simulink model "DR18E_Testpult"  (R2017a)
settings: Solver=ode1  StartTime=0.0  StopTime=Inf  FixedStep=0.001  RelTol=1e-3
PostLoadFcn:
  | , if any(exist('dsrtsu_mdlpostloadfcn', 'file') == [2, 3, 6]), try dsrtsu_mdlpostloadfcn('Execute', bdroot); catch fprintf('Error in PostLoadFcn (dsrtsu_mdlpostloadfcn) for model "%s":\n %s\n', bdroot, lasterr); end, end,
model workspace: external: MATLAB File C:\Users\DeltaRacing\Documents\dSPACE\MABX_DR18E\Model\DR18E_MABX_Parameter.m (data not in the file)
values from neighbouring files (symbols this model uses):
  am = 1/Ts    (= 1)    [DR18E_MABX_Parameter.m]
  bm = K/Ts    (= 0.05)    [DR18E_MABX_Parameter.m]
  cf = 41350    [DR18E_MABX_Parameter.m]
  cr = 41350    [DR18E_MABX_Parameter.m]
  Derating_HV_Battery_Kapa = 1    [DR18E_MABX_Parameter.m]
  Derating_Start_km = 16    [DR18E_MABX_Parameter.m]
  Drive_Mode = 0    [DR18E_MABX_Parameter.m]
  g = 1    [DR18E_MABX_Parameter.m]
  Gas_Modus = 2    [DR18E_MABX_Parameter.m]
  HV_Power_max = 80    [DR18E_MABX_Parameter.m]
  i_Getriebe = 3.3    [DR18E_MABX_Parameter.m]
  i_Lenkgetriebe = 4.32    [DR18E_MABX_Parameter.m]
  K_SET = 1    [DR18E_MABX_Parameter.m]
  Kapazitaet_HV_Battery_kWh = 6.6    [DR18E_MABX_Parameter.m]
  KW_T_Soll = 37    [DR18E_MABX_Parameter.m]
  lf = 1.2    [DR18E_MABX_Parameter.m]
  lr = 1.15    [DR18E_MABX_Parameter.m]
  m = 310    [DR18E_MABX_Parameter.m]
  M_max = 150    [DR18E_MABX_Parameter.m]
  Power_Limit_onoff = 0    [DR18E_MABX_Parameter.m]
  Reifenradius = 0.2351    [DR18E_MABX_Parameter.m]
  Strecke_Endu_km = 22    [DR18E_MABX_Parameter.m]
  TC_Decr_Gas = 0.00005    (= 5e-05)    [DR18E_MABX_Parameter.m]
  TC_Derivative = 0.4    [DR18E_MABX_Parameter.m]
  TC_Incr_Gas = 0.005    [DR18E_MABX_Parameter.m]
  TC_On = 0    [DR18E_MABX_Parameter.m]
  TC_Relay_Off = 0.065    [DR18E_MABX_Parameter.m]
  TC_Relay_On = 0.07    [DR18E_MABX_Parameter.m]
  TV_Mode = 2    [DR18E_MABX_Parameter.m]
  TV_On = 0    [DR18E_MABX_Parameter.m]
  TV_Override = 1    [DR18E_MABX_Parameter.m]
  y = 0.8    [DR18E_MABX_Parameter.m]
undefined symbols (not defined in the file or in its folder): D, DiscIntNeverNeededParam, I, K_OL, P
libraries: simulink x288, rtican x105, rtiusbflightreclib x40, rti1401lib_dio_type3 x10, simulink_extras x10, rti1401lib_adc_type4 x8, rti1401lib_II_base x7
(part 9 of 28)

== system DR18E_Testpult/Eingabe Fahrzeug/Sensorboard Mitte ==
  Bus Creator : BusCreator  Inputs=4
  Bus Creator1 : BusCreator  Inputs=3
  Dashboard_AUX : rtican/RTICAN Receive (RX)   Reserved1=[]  Reserved2=[]  Reserved3=[]  Reserved4=[]  SfcnMessage=[]  Msg_Struct=[]  BoardTypeNo=[]  BoardNo=[]  ChannelNo=[]  Parameters=[]  DialogFcn=[]  UnitName=[]  Revision=[]  UnitValues=[]  DSProperties=struct('RTI',struct('Version',uint32(5),'BlockType',struct('isSLSource',uint8(1),'isSLSink',uint8(1),'isHWSource',uint8(0),'isHWSink',uint8(0),'isSetup',uint8(0),'isInline',uint8(1),'isNonInline',uint8(0),'isInterrupt',uint8(0),'isChannelwise',uint8(0)),'IOBoardType','RTICAN','UnitType','MESSAGE','Identifier','RX','DialogType','MSVC','BlockSet','RTICAN','SlaveProcessor','CAN'))  RTIBlockInterface=struct('OutputPortsWidth',int32([1 1 1 1 1]),'OutputPortsActive',[1 1 1 1 1],'OutputPortsName',{{'Notaus_Cockpit','Crashsensor',['RX status'],['RX time'],['RX delta time']}},'OutputPortsDataType',{{'SS_DOUBLE','SS_DOUBLE','SS_DOUBLE','SS_DOUBLE','SS_DOUBLE'}},'OutputPortsLabel',{{'Notaus_Cockpit','Crashsensor','','',''}},'OutputPortsLabelMode','ON','InputPortsWidth',int32(0),'InputPortsActive',0,'DialogFcn','rtican_message_interface_gui','BlockDisplay',{{'','center'}},'IconTransparency','on','ParameterTunableNames',{{}},'InitLevel',3,'BlockName',struct('Token',{{'Dashboard_AUX'}}),'SampleTime',{{-1}},'TriggerPort',{{'none'}},'EnablePort',{{'none'}})  RTIBlockParameters=struct('BoardTypeNo',{{1,'OFF',[]}},'BoardNo',{{2,'ON',[1 16]}},'ChannelNo',{{1,'ON',[1 2]}},'Parameters',{{struct('DataFileSupport',struct('DataFileSelectedMaster',1,'DataFileSelectedLocal',1,'DataFileName','c:\users\deltaracing\documents\canoe\dr18e\dbc\dr18e.dbc|','DataFileDate',['16-Feb-2019 13:23:09'],'SelectedFile','..\..\..\canoe\dr18e_test\dr18e\dbc\dr18e.dbc','InterfaceFcn','rtican_dbc_file_parser'),'Options',struct('StatusSelected',1,'TimeSelected',1,'DeltaTimeSelected',1,'BytePortSelected',0,'MessageLengthSelected',0,'TriggerPort',struct('Selected',0,'TriggerType',0),'UserCoding',struct('Selected',0,'InterfaceFile','UserDecodingFile','FcnName','UserDecodeFcn','InportSelected',0,'InportWidth',1,'OutportSelected',0,'OutportWidth',1),'EnablePortSelected',0,'SignalOnPortnameSelected',1,'UseRXService',0),'Message',struct('MsgOnBlocknameSelected',1,'MsgName','Dashboard_AUX','MsgIdFormat',0,'MsgId',786,'MsgLength',2,'NumSignals',2,'SampleTime',-1,'Signal',struct('SgnName',{'Notaus_Cockpit','Crashsensor'},'SgnStartBit',{0,8},'SgnLength',{8,8},'ByteLayout',{0,0},'Factor',{1,1},'Offset',{0,0},'SgnComment',{'',''},'SgnUnit',{'',''},'Min',{0,0},'Max',{255,255},'SgnType',{0,0},'SLDataType',{'SS_DOUBLE','SS_DOUBLE'},'DataType',{0,0},'ModeValue',{-1,-1}),'MsgIdNumFormat',0,'MsgComment',{{''}}),'Version',1.2,'general',struct('isFromLib',0)),'OFF',[]}},'GroupId',{{struct('Group',{{'RTICAN'}},'No',1,'Behavior',{{'NAMECHANGE'}},'BlockType',{{'SINK'}},'NameChangeFlag',0),'OFF',[]}},'SFcnRTICANMessage',{{struct('MsgType','RX','SFcnPortType','Scalar','MsgName','Dashboard_AUX','MsgIdFormat','STD','MsgId',786,'MsgLength',2,'NumSignals',2,'SampleTime',-1,'Signal',struct('SgnName',{'Notaus_Cockpit','Crashsensor'},'SgnStartBit',{0,8},'SgnLength',{8,8},'ByteLayout',{['little endian'],['little endian']},'Factor',{1,1},'Offset',{0,0},'SgnType',{'standard','standard'},'SLDataType',{'SS_DOUBLE','SS_DOUBLE'},'DataType',{['unsigned int'],['unsigned int']},'ModeValue',{-1,-1}),'StatusSelected','yes','TimeSelected','yes','DeltaTimeSelected','yes','BytePortSelected','no','MessageLengthSelected','no','TriggerPort',struct('Selected','no','TriggerType',0),'UserCoding',struct('Selected','no','InterfaceFile','UserDecodingFile','FcnName','UserDecodeFcn','InportSelected','no','InportWidth',1,'OutportSelected','no','OutportWidth',1),'EnablePortSelected','no','UseRXService','no','BoardType','DS1','BoardNo',2,'ControllerNo',1),'OFF',[]}},'TLCFileName',{{'rtican_rx_message','OFF',[]}})  RTISFcnParameters=struct('SFcnRTICANMessage','struct','TLCFileName','char')  RTIBlockParaDefault=struct('BoardTypeNo',4302,'BoardNo',1,'ChannelNo',1,'Parameters',struct('DataFileSupport',struct('DataFileSelectedMaster',0,'DataFileSelectedLocal',0,'DataFileName','','DataFileDate','','SelectedFile',['<no file selected>']),'Options',struct('StatusSelected',1,'TimeSelected',1,'DeltaTimeSelected',1,'BytePortSelected',0,'MessageLengthSelected',0,'TriggerPort',struct('Selected',0,'TriggerType','rising'),'UserCoding',struct('Selected',0,'InterfaceFile','UserDecodingFile','FcnName','UserDecodeFcn','InportSelected',0,'InportWidth',1,'OutportSelected',0,'OutportWidth',1),'EnablePortSelected',0,'SignalOnPortnameSelected',1,'UseRXService',0),'Message',struct('MsgOnBlocknameSelected',0,'MsgName',['RX Message'],'MsgIdFormat',0,'MsgId',100,'MsgLength',8,'NumSignals',1,'SampleTime',-1,'Signal',struct('SgnName',['RX signal'],'SgnStartBit',0,'SgnLength',8,'SgnType',0,'ModeValue',-1,'DataType',0,'SLDataType','SS_DOUBLE','ByteLayout',0,'Factor',1,'Offset',0,'Min',0,'Max',255,'SgnComment',{{}},'SgnUnit',''),'MsgIdNumFormat',0,'MsgComment',{{''}}),'Version',1.2,'general',struct('isFromLib',1)),'GroupId',struct('Group',{{'RTICAN'}},'No',1,'Behavior',{{'NAMECHANGE'}},'BlockType',{{'SINK'}},'NameChangeFlag',0),'SFcnRTICANMessage',struct('MsgType','RX','MsgName',['RX Message'],'MsgIdFormat','STD','MsgId',100,'MsgLength',8,'NumSignals',1,'SampleTime',-1,'Signal',struct('SgnName',['RX signal'],'SgnStartBit',0,'SgnLength',8,'SgnType','standard','ModeValue',-1,'DataType',['unsigned int'],'ByteLayout',['little endian'],'SLDataType','SS_DOUBLE','Factor',1,'Offset',0),'StatusSelected','yes','TimeSelected','yes','DeltaTimeSelected','yes','BytePortSelected','no','MessageLengthSelected','no','EnablePortSelected','no','UserCoding',struct('Selected','no','InterfaceFile','UserDecodingFile','FcnName','UserDecodeFcn','InportSelected','no','InportWidth',1,'OutportSelected','no','OutportWidth',1),'TriggerPort',struct('Selected','no','TriggerType','rising'),'UseRXService','no','BoardType','DS4302','BoardNo',1,'ControllerNo',1,'SFcnPortType','Scalar'),'TLCFileName','rtican_rx_message')
      settings: AttributesFormatString=Group Id: RTICAN1\n  SourceProductName=dSPACE RTI CAN Blockset
  Dashboard_Buttons : rtican/RTICAN Receive (RX)   Reserved1=[]  Reserved2=[]  Reserved3=[]  Reserved4=[]  SfcnMessage=[]  Msg_Struct=[]  BoardTypeNo=[]  BoardNo=[]  ChannelNo=[]  Parameters=[]  DialogFcn=[]  UnitName=[]  Revision=[]  UnitValues=[]  DSProperties=struct('RTI',struct('Version',uint32(5),'BlockType',struct('isSLSource',uint8(1),'isSLSink',uint8(1),'isHWSource',uint8(0),'isHWSink',uint8(0),'isSetup',uint8(0),'isInline',uint8(1),'isNonInline',uint8(0),'isInterrupt',uint8(0),'isChannelwise',uint8(0)),'IOBoardType','RTICAN','UnitType','MESSAGE','Identifier','RX','DialogType','MSVC','BlockSet','RTICAN','SlaveProcessor','CAN'))  RTIBlockInterface=struct('OutputPortsWidth',int32([1 1 1 1]),'OutputPortsActive',[1 1 1 1],'OutputPortsName',{{'Starttaster',['RX status'],['RX time'],['RX delta time']}},'OutputPortsDataType',{{'SS_DOUBLE','SS_DOUBLE','SS_DOUBLE','SS_DOUBLE'}},'OutputPortsLabel',{{'Starttaster','','',''}},'OutputPortsLabelMode','ON','InputPortsWidth',int32(0),'InputPortsActive',0,'DialogFcn','rtican_message_interface_gui','BlockDisplay',{{'','center'}},'IconTransparency','on','ParameterTunableNames',{{}},'InitLevel',3,'BlockName',struct('Token',{{'Dashboard_Buttons'}}),'SampleTime',{{-1}},'TriggerPort',{{'none'}},'EnablePort',{{'none'}})  RTIBlockParameters=struct('BoardTypeNo',{{1,'OFF',[]}},'BoardNo',{{2,'ON',[1 16]}},'ChannelNo',{{1,'ON',[1 2]}},'Parameters',{{struct('DataFileSupport',struct('DataFileSelectedMaster',1,'DataFileSelectedLocal',1,'DataFileName','c:\users\deltaracing\documents\canoe\dr18e\dbc\dr18e.dbc|','DataFileDate',['16-Feb-2019 13:23:09'],'SelectedFile','..\..\..\canoe\dr18e_test\dr18e\dbc\dr18e.dbc','InterfaceFcn','rtican_dbc_file_parser'),'Options',struct('StatusSelected',1,'TimeSelected',1,'DeltaTimeSelected',1,'BytePortSelected',0,'MessageLengthSelected',0,'TriggerPort',struct('Selected',0,'TriggerType',0),'UserCoding',struct('Selected',0,'InterfaceFile','UserDecodingFile','FcnName','UserDecodeFcn','InportSelected',0,'InportWidth',1,'OutportSelected',0,'OutportWidth',1),'EnablePortSelected',0,'SignalOnPortnameSelected',1,'UseRXService',0),'Message',struct('MsgOnBlocknameSelected',1,'MsgName','Dashboard_Buttons','MsgIdFormat',0,'MsgId',787,'MsgLength',1,'NumSignals',1,'SampleTime',-1,'Signal',struct('SgnName','Starttaster','SgnStartBit',0,'SgnLength',8,'ByteLayout',0,'Factor',1,'Offset',0,'SgnComment','','SgnUnit','','Min',0,'Max',255,'SgnType',0,'SLDataType','SS_DOUBLE','DataType',0,'ModeValue',-1),'MsgIdNumFormat',0,'MsgComment',{{''}}),'Version',1.2,'general',struct('isFromLib',0)),'OFF',[]}},'GroupId',{{struct('Group',{{'RTICAN'}},'No',1,'Behavior',{{'NAMECHANGE'}},'BlockType',{{'SINK'}},'NameChangeFlag',0),'OFF',[]}},'SFcnRTICANMessage',{{struct('MsgType','RX','SFcnPortType','Scalar','MsgName','Dashboard_Buttons','MsgIdFormat','STD','MsgId',787,'MsgLength',1,'NumSignals',1,'SampleTime',-1,'Signal',struct('SgnName','Starttaster','SgnStartBit',0,'SgnLength',8,'ByteLayout',['little endian'],'Factor',1,'Offset',0,'SgnType','standard','SLDataType','SS_DOUBLE','DataType',['unsigned int'],'ModeValue',-1),'StatusSelected','yes','TimeSelected','yes','DeltaTimeSelected','yes','BytePortSelected','no','MessageLengthSelected','no','TriggerPort',struct('Selected','no','TriggerType',0),'UserCoding',struct('Selected','no','InterfaceFile','UserDecodingFile','FcnName','UserDecodeFcn','InportSelected','no','InportWidth',1,'OutportSelected','no','OutportWidth',1),'EnablePortSelected','no','UseRXService','no','BoardType','DS1','BoardNo',2,'ControllerNo',1),'OFF',[]}},'TLCFileName',{{'rtican_rx_message','OFF',[]}})  RTISFcnParameters=struct('SFcnRTICANMessage','struct','TLCFileName','char')  RTIBlockParaDefault=struct('BoardTypeNo',4302,'BoardNo',1,'ChannelNo',1,'Parameters',struct('DataFileSupport',struct('DataFileSelectedMaster',0,'DataFileSelectedLocal',0,'DataFileName','','DataFileDate','','SelectedFile',['<no file selected>']),'Options',struct('StatusSelected',1,'TimeSelected',1,'DeltaTimeSelected',1,'BytePortSelected',0,'MessageLengthSelected',0,'TriggerPort',struct('Selected',0,'TriggerType','rising'),'UserCoding',struct('Selected',0,'InterfaceFile','UserDecodingFile','FcnName','UserDecodeFcn','InportSelected',0,'InportWidth',1,'OutportSelected',0,'OutportWidth',1),'EnablePortSelected',0,'SignalOnPortnameSelected',1,'UseRXService',0),'Message',struct('MsgOnBlocknameSelected',0,'MsgName',['RX Message'],'MsgIdFormat',0,'MsgId',100,'MsgLength',8,'NumSignals',1,'SampleTime',-1,'Signal',struct('SgnName',['RX signal'],'SgnStartBit',0,'SgnLength',8,'SgnType',0,'ModeValue',-1,'DataType',0,'SLDataType','SS_DOUBLE','ByteLayout',0,'Factor',1,'Offset',0,'Min',0,'Max',255,'SgnComment',{{}},'SgnUnit',''),'MsgIdNumFormat',0,'MsgComment',{{''}}),'Version',1.2,'general',struct('isFromLib',1)),'GroupId',struct('Group',{{'RTICAN'}},'No',1,'Behavior',{{'NAMECHANGE'}},'BlockType',{{'SINK'}},'NameChangeFlag',0),'SFcnRTICANMessage',struct('MsgType','RX','MsgName',['RX Message'],'MsgIdFormat','STD','MsgId',100,'MsgLength',8,'NumSignals',1,'SampleTime',-1,'Signal',struct('SgnName',['RX signal'],'SgnStartBit',0,'SgnLength',8,'SgnType','standard','ModeValue',-1,'DataType',['unsigned int'],'ByteLayout',['little endian'],'SLDataType','SS_DOUBLE','Factor',1,'Offset',0),'StatusSelected','yes','TimeSelected','yes','DeltaTimeSelected','yes','BytePortSelected','no','MessageLengthSelected','no','EnablePortSelected','no','UserCoding',struct('Selected','no','InterfaceFile','UserDecodingFile','FcnName','UserDecodeFcn','InportSelected','no','InportWidth',1,'OutportSelected','no','OutportWidth',1),'TriggerPort',struct('Selected','no','TriggerType','rising'),'UseRXService','no','BoardType','DS4302','BoardNo',1,'ControllerNo',1,'SFcnPortType','Scalar'),'TLCFileName','rtican_rx_message')
      settings: AttributesFormatString=Group Id: RTICAN1\n  SourceProductName=dSPACE RTI CAN Blockset
  DrehzahlTimeout : Constant  Value=1100
  Gain : Gain  Gain=1/255
  Gain1 : Gain  Gain=1/255
  Gain2 : Gain  Gain=1/255
  RPM_Front : rtican/RTICAN Receive (RX)   Reserved1=[]  Reserved2=[]  Reserved3=[]  Reserved4=[]  SfcnMessage=[]  Msg_Struct=[]  BoardTypeNo=[]  BoardNo=[]  ChannelNo=[]  Parameters=[]  DialogFcn=[]  UnitName=[]  Revision=[]  UnitValues=[]  DSProperties=struct('RTI',struct('Version',uint32(5),'BlockType',struct('isSLSource',uint8(1),'isSLSink',uint8(1),'isHWSource',uint8(0),'isHWSink',uint8(0),'isSetup',uint8(0),'isInline',uint8(1),'isNonInline',uint8(0),'isInterrupt',uint8(0),'isChannelwise',uint8(0)),'IOBoardType','RTICAN','UnitType','MESSAGE','Identifier','RX','DialogType','MSVC','BlockSet','RTICAN','SlaveProcessor','CAN'))  RTIBlockInterface=struct('OutputPortsWidth',int32([1 1 1 1 1]),'OutputPortsActive',[1 1 1 1 1],'OutputPortsName',{{'RPM_Left','RPM_Right',['RX status'],['RX time'],['RX delta time']}},'OutputPortsDataType',{{'SS_DOUBLE','SS_DOUBLE','SS_DOUBLE','SS_DOUBLE','SS_DOUBLE'}},'OutputPortsLabel',{{'RPM_Left','RPM_Right','','',''}},'OutputPortsLabelMode','ON','InputPortsWidth',int32(0),'InputPortsActive',0,'DialogFcn','rtican_message_interface_gui','BlockDisplay',{{'','center'}},'IconTransparency','on','ParameterTunableNames',{{}},'InitLevel',3,'BlockName',struct('Token',{{'RPM_Front'}}),'SampleTime',{{-1}},'TriggerPort',{{'none'}},'EnablePort',{{'none'}})  RTIBlockParameters=struct('BoardTypeNo',{{1,'OFF',[]}},'BoardNo',{{2,'ON',[1 16]}},'ChannelNo',{{1,'ON',[1 2]}},'Parameters',{{struct('DataFileSupport',struct('DataFileSelectedMaster',1,'DataFileSelectedLocal',1,'DataFileName','c:\users\deltaracing\documents\canoe\dr18e\dbc\dr18e.dbc|','DataFileDate',['16-Feb-2019 13:23:09'],'SelectedFile','..\..\..\canoe\dr18e_test\dr18e\dbc\dr18e.dbc','InterfaceFcn','rtican_dbc_file_parser'),'Options',struct('StatusSelected',1,'TimeSelected',1,'DeltaTimeSelected',1,'BytePortSelected',0,'MessageLengthSelected',0,'TriggerPort',struct('Selected',0,'TriggerType',0),'UserCoding',struct('Selected',0,'InterfaceFile','UserDecodingFile','FcnName','UserDecodeFcn','InportSelected',0,'InportWidth',1,'OutportSelected',0,'OutportWidth',1),'EnablePortSelected',0,'SignalOnPortnameSelected',1,'UseRXService',0),'Message',struct('MsgOnBlocknameSelected',1,'MsgName','RPM_Front','MsgIdFormat',0,'MsgId',291,'MsgLength',4,'NumSignals',2,'SampleTime',-1,'Signal',struct('SgnName',{'RPM_Left','RPM_Right'},'SgnStartBit',{0,16},'SgnLength',{16,16},'ByteLayout',{0,0},'Factor',{1,1},'Offset',{0,0},'SgnComment',{'',''},'SgnUnit',{'U/min','U/min'},'Min',{0,0},'Max',{1500,1500},'SgnType',{0,0},'SLDataType',{'SS_DOUBLE','SS_DOUBLE'},'DataType',{0,0},'ModeValue',{-1,-1}),'MsgIdNumFormat',0,'MsgComment',{{''}}),'Version',1.2,'general',struct('isFromLib',0)),'OFF',[]}},'GroupId',{{struct('Group',{{'RTICAN'}},'No',1,'Behavior',{{'NAMECHANGE'}},'BlockType',{{'SINK'}},'NameChangeFlag',0),'OFF',[]}},'SFcnRTICANMessage',{{struct('MsgType','RX','SFcnPortType','Scalar','MsgName','RPM_Front','MsgIdFormat','STD','MsgId',291,'MsgLength',4,'NumSignals',2,'SampleTime',-1,'Signal',struct('SgnName',{'RPM_Left','RPM_Right'},'SgnStartBit',{0,16},'SgnLength',{16,16},'ByteLayout',{['little endian'],['little endian']},'Factor',{1,1},'Offset',{0,0},'SgnType',{'standard','standard'},'SLDataType',{'SS_DOUBLE','SS_DOUBLE'},'DataType',{['unsigned int'],['unsigned int']},'ModeValue',{-1,-1}),'StatusSelected','yes','TimeSelected','yes','DeltaTimeSelected','yes','BytePortSelected','no','MessageLengthSelected','no','TriggerPort',struct('Selected','no','TriggerType',0),'UserCoding',struct('Selected','no','InterfaceFile','UserDecodingFile','FcnName','UserDecodeFcn','InportSelected','no','InportWidth',1,'OutportSelected','no','OutportWidth',1),'EnablePortSelected','no','UseRXService','no','BoardType','DS1','BoardNo',2,'ControllerNo',1),'OFF',[]}},'TLCFileName',{{'rtican_rx_message','OFF',[]}})  RTISFcnParameters=struct('SFcnRTICANMessage','struct','TLCFileName','char')  RTIBlockParaDefault=struct('BoardTypeNo',4302,'BoardNo',1,'ChannelNo',1,'Parameters',struct('DataFileSupport',struct('DataFileSelectedMaster',0,'DataFileSelectedLocal',0,'DataFileName','','DataFileDate','','SelectedFile',['<no file selected>']),'Options',struct('StatusSelected',1,'TimeSelected',1,'DeltaTimeSelected',1,'BytePortSelected',0,'MessageLengthSelected',0,'TriggerPort',struct('Selected',0,'TriggerType','rising'),'UserCoding',struct('Selected',0,'InterfaceFile','UserDecodingFile','FcnName','UserDecodeFcn','InportSelected',0,'InportWidth',1,'OutportSelected',0,'OutportWidth',1),'EnablePortSelected',0,'SignalOnPortnameSelected',1,'UseRXService',0),'Message',struct('MsgOnBlocknameSelected',0,'MsgName',['RX Message'],'MsgIdFormat',0,'MsgId',100,'MsgLength',8,'NumSignals',1,'SampleTime',-1,'Signal',struct('SgnName',['RX signal'],'SgnStartBit',0,'SgnLength',8,'SgnType',0,'ModeValue',-1,'DataType',0,'SLDataType','SS_DOUBLE','ByteLayout',0,'Factor',1,'Offset',0,'Min',0,'Max',255,'SgnComment',{{}},'SgnUnit',''),'MsgIdNumFormat',0,'MsgComment',{{''}}),'Version',1.2,'general',struct('isFromLib',1)),'GroupId',struct('Group',{{'RTICAN'}},'No',1,'Behavior',{{'NAMECHANGE'}},'BlockType',{{'SINK'}},'NameChangeFlag',0),'SFcnRTICANMessage',struct('MsgType','RX','MsgName',['RX Message'],'MsgIdFormat','STD','MsgId',100,'MsgLength',8,'NumSignals',1,'SampleTime',-1,'Signal',struct('SgnName',['RX signal'],'SgnStartBit',0,'SgnLength',8,'SgnType','standard','ModeValue',-1,'DataType',['unsigned int'],'ByteLayout',['little endian'],'SLDataType','SS_DOUBLE','Factor',1,'Offset',0),'StatusSelected','yes','TimeSelected','yes','DeltaTimeSelected','yes','BytePortSelected','no','MessageLengthSelected','no','EnablePortSelected','no','UserCoding',struct('Selected','no','InterfaceFile','UserDecodingFile','FcnName','UserDecodeFcn','InportSelected','no','InportWidth',1,'OutportSelected','no','OutportWidth',1),'TriggerPort',struct('Selected','no','TriggerType','rising'),'UseRXService','no','BoardType','DS4302','BoardNo',1,'ControllerNo',1,'SFcnPortType','Scalar'),'TLCFileName','rtican_rx_message')
      settings: AttributesFormatString=Group Id: RTICAN1\n  SourceProductName=dSPACE RTI CAN Blockset
  RX Timeout Detection : Subsystem
  Terminator_6 : Terminator
  Terminator_7 : Terminator
  Transmit OK Detection3 : Subsystem
  Transmit OK Detection4 : Subsystem
  SensorboardMitteOut : Outport
  wires:
  Transmit OK Detection3/1(TX Warn) -> Terminator_6/1
  Dashboard_AUX/5 -> Transmit OK Detection3/2(TX delta time)
  Dashboard_AUX/3 -> Transmit OK Detection3/1(TX status)
  Transmit OK Detection4/1(TX Warn) -> Terminator_7/1
  Dashboard_Buttons/4 -> Transmit OK Detection4/2(TX delta time)
  Dashboard_Buttons/2 -> Transmit OK Detection4/1(TX status)
  Bus Creator/1 -> SensorboardMitteOut/1  "RX_SensorboardMitte"
  Bus Creator1/1 -> Bus Creator/4  "Drehzahlen vorne"
  DrehzahlTimeout/1 -> RX Timeout Detection/2(Timeout (n Samples))
  RPM_Front/3 -> RX Timeout Detection/1(RX status)
  RX Timeout Detection/1(RX Timeout Error) -> Bus Creator1/3  "RX Timeout Error"
  Gain/1 -> Bus Creator/1  "Notaus_Cockpit"
  Gain1/1 -> Bus Creator/2  "Crashsensor"
  Gain2/1 -> Bus Creator/3  "Starttaster"
  Dashboard_AUX/1 -> Gain/1  "Notaus_Cockpit"
  Dashboard_AUX/2 -> Gain1/1  "Crashsensor"
  Dashboard_Buttons/1 -> Gain2/1  "Starttaster"
  RPM_Front/1 -> Bus Creator1/1  "RPM_Left"
  RPM_Front/2 -> Bus Creator1/2  "RPM_Right"

== system DR18E_Testpult/Eingabe Fahrzeug/Sensorboard Rear ==
  Bus Creator : BusCreator  Inputs=5
  ES_rear : rtican/RTICAN Receive (RX)   Reserved1=[]  Reserved2=[]  Reserved3=[]  Reserved4=[]  SfcnMessage=[]  Msg_Struct=[]  BoardTypeNo=[]  BoardNo=[]  ChannelNo=[]  Parameters=[]  DialogFcn=[]  UnitName=[]  Revision=[]  UnitValues=[]  DSProperties=struct('RTI',struct('Version',uint32(5),'BlockType',struct('isSLSource',uint8(1),'isSLSink',uint8(1),'isHWSource',uint8(0),'isHWSink',uint8(0),'isSetup',uint8(0),'isInline',uint8(1),'isNonInline',uint8(0),'isInterrupt',uint8(0),'isChannelwise',uint8(0)),'IOBoardType','RTICAN','UnitType','MESSAGE','Identifier','RX','DialogType','MSVC','BlockSet','RTICAN','SlaveProcessor','CAN'))  RTIBlockInterface=struct('OutputPortsWidth',int32([1 1 1 1 1]),'OutputPortsActive',[1 1 1 1 1],'OutputPortsName',{{'Notaus_links','Notaus_rechts',['RX status'],['RX time'],['RX delta time']}},'OutputPortsDataType',{{'SS_DOUBLE','SS_DOUBLE','SS_DOUBLE','SS_DOUBLE','SS_DOUBLE'}},'OutputPortsLabel',{{'Notaus_links','Notaus_rechts','','',''}},'OutputPortsLabelMode','ON','InputPortsWidth',int32(0),'InputPortsActive',0,'DialogFcn','rtican_message_interface_gui','BlockDisplay',{{'','center'}},'IconTransparency','on','ParameterTunableNames',{{}},'InitLevel',3,'BlockName',struct('Token',{{'ES_rear'}}),'SampleTime',{{-1}},'TriggerPort',{{'none'}},'EnablePort',{{'none'}})  RTIBlockParameters=struct('BoardTypeNo',{{1,'OFF',[]}},'BoardNo',{{2,'ON',[1 16]}},'ChannelNo',{{1,'ON',[1 2]}},'Parameters',{{struct('DataFileSupport',struct('DataFileSelectedMaster',1,'DataFileSelectedLocal',1,'DataFileName','c:\users\deltaracing\documents\canoe\dr18e\dbc\dr18e.dbc|','DataFileDate',['16-Feb-2019 13:23:09'],'SelectedFile','..\..\..\canoe\dr18e_test\dr18e\dbc\dr18e.dbc','InterfaceFcn','rtican_dbc_file_parser'),'Options',struct('StatusSelected',1,'TimeSelected',1,'DeltaTimeSelected',1,'BytePortSelected',0,'MessageLengthSelected',0,'TriggerPort',struct('Selected',0,'TriggerType',0),'UserCoding',struct('Selected',0,'InterfaceFile','UserDecodingFile','FcnName','UserDecodeFcn','InportSelected',0,'InportWidth',1,'OutportSelected',0,'OutportWidth',1),'EnablePortSelected',0,'SignalOnPortnameSelected',1,'UseRXService',0),'Message',struct('MsgOnBlocknameSelected',1,'MsgName','ES_rear','MsgIdFormat',0,'MsgId',789,'MsgLength',2,'NumSignals',2,'SampleTime',-1,'Signal',struct('SgnName',{'Notaus_links','Notaus_rechts'},'SgnStartBit',{0,8},'SgnLength',{8,8},'ByteLayout',{0,0},'Factor',{1,1},'Offset',{0,0},'SgnComment',{'',''},'SgnUnit',{'',''},'Min',{0,0},'Max',{0,0},'SgnType',{0,0},'SLDataType',{'SS_DOUBLE','SS_DOUBLE'},'DataType',{0,0},'ModeValue',{-1,-1}),'MsgIdNumFormat',0,'MsgComment',{{''}}),'Version',1.2,'general',struct('isFromLib',0)),'OFF',[]}},'GroupId',{{struct('Group',{{'RTICAN'}},'No',1,'Behavior',{{'NAMECHANGE'}},'BlockType',{{'SINK'}},'NameChangeFlag',0),'OFF',[]}},'SFcnRTICANMessage',{{struct('MsgType','RX','SFcnPortType','Scalar','MsgName','ES_rear','MsgIdFormat','STD','MsgId',789,'MsgLength',2,'NumSignals',2,'SampleTime',-1,'Signal',struct('SgnName',{'Notaus_links','Notaus_rechts'},'SgnStartBit',{0,8},'SgnLength',{8,8},'ByteLayout',{['little endian'],['little endian']},'Factor',{1,1},'Offset',{0,0},'SgnType',{'standard','standard'},'SLDataType',{'SS_DOUBLE','SS_DOUBLE'},'DataType',{['unsigned int'],['unsigned int']},'ModeValue',{-1,-1}),'StatusSelected','yes','TimeSelected','yes','DeltaTimeSelected','yes','BytePortSelected','no','MessageLengthSelected','no','TriggerPort',struct('Selected','no','TriggerType',0),'UserCoding',struct('Selected','no','InterfaceFile','UserDecodingFile','FcnName','UserDecodeFcn','InportSelected','no','InportWidth',1,'OutportSelected','no','OutportWidth',1),'EnablePortSelected','no','UseRXService','no','BoardType','DS1','BoardNo',2,'ControllerNo',1),'OFF',[]}},'TLCFileName',{{'rtican_rx_message','OFF',[]}})  RTISFcnParameters=struct('SFcnRTICANMessage','struct','TLCFileName','char')  RTIBlockParaDefault=struct('BoardTypeNo',4302,'BoardNo',1,'ChannelNo',1,'Parameters',struct('DataFileSupport',struct('DataFileSelectedMaster',0,'DataFileSelectedLocal',0,'DataFileName','','DataFileDate','','SelectedFile',['<no file selected>']),'Options',struct('StatusSelected',1,'TimeSelected',1,'DeltaTimeSelected',1,'BytePortSelected',0,'MessageLengthSelected',0,'TriggerPort',struct('Selected',0,'TriggerType','rising'),'UserCoding',struct('Selected',0,'InterfaceFile','UserDecodingFile','FcnName','UserDecodeFcn','InportSelected',0,'InportWidth',1,'OutportSelected',0,'OutportWidth',1),'EnablePortSelected',0,'SignalOnPortnameSelected',1,'UseRXService',0),'Message',struct('MsgOnBlocknameSelected',0,'MsgName',['RX Message'],'MsgIdFormat',0,'MsgId',100,'MsgLength',8,'NumSignals',1,'SampleTime',-1,'Signal',struct('SgnName',['RX signal'],'SgnStartBit',0,'SgnLength',8,'SgnType',0,'ModeValue',-1,'DataType',0,'SLDataType','SS_DOUBLE','ByteLayout',0,'Factor',1,'Offset',0,'Min',0,'Max',255,'SgnComment',{{}},'SgnUnit',''),'MsgIdNumFormat',0,'MsgComment',{{''}}),'Version',1.2,'general',struct('isFromLib',1)),'GroupId',struct('Group',{{'RTICAN'}},'No',1,'Behavior',{{'NAMECHANGE'}},'BlockType',{{'SINK'}},'NameChangeFlag',0),'SFcnRTICANMessage',struct('MsgType','RX','MsgName',['RX Message'],'MsgIdFormat','STD','MsgId',100,'MsgLength',8,'NumSignals',1,'SampleTime',-1,'Signal',struct('SgnName',['RX signal'],'SgnStartBit',0,'SgnLength',8,'SgnType','standard','ModeValue',-1,'DataType',['unsigned int'],'ByteLayout',['little endian'],'SLDataType','SS_DOUBLE','Factor',1,'Offset',0),'StatusSelected','yes','TimeSelected','yes','DeltaTimeSelected','yes','BytePortSelected','no','MessageLengthSelected','no','EnablePortSelected','no','UserCoding',struct('Selected','no','InterfaceFile','UserDecodingFile','FcnName','UserDecodeFcn','InportSelected','no','InportWidth',1,'OutportSelected','no','OutportWidth',1),'TriggerPort',struct('Selected','no','TriggerType','rising'),'UseRXService','no','BoardType','DS4302','BoardNo',1,'ControllerNo',1,'SFcnPortType','Scalar'),'TLCFileName','rtican_rx_message')
      settings: AttributesFormatString=Group Id: RTICAN1\n  SourceProductName=dSPACE RTI CAN Blockset
  FlightRecorder1 : Subsystem
  FlightRecorder2 : Subsystem
  FlightRecorder3 : Subsystem
  Gain : Gain  Gain=1/255
  Gain1 : Gain  Gain=1/255
  Oiltemperature : rtican/RTICAN Receive (RX)   Reserved1=[]  Reserved2=[]  Reserved3=[]  Reserved4=[]  SfcnMessage=[]  Msg_Struct=[]  BoardTypeNo=[]  BoardNo=[]  ChannelNo=[]  Parameters=[]  DialogFcn=[]  UnitName=[]  Revision=[]  UnitValues=[]  DSProperties=struct('RTI',struct('Version',uint32(5),'BlockType',struct('isSLSource',uint8(1),'isSLSink',uint8(1),'isHWSource',uint8(0),'isHWSink',uint8(0),'isSetup',uint8(0),'isInline',uint8(1),'isNonInline',uint8(0),'isInterrupt',uint8(0),'isChannelwise',uint8(0)),'IOBoardType','RTICAN','UnitType','MESSAGE','Identifier','RX','DialogType','MSVC','BlockSet','RTICAN','SlaveProcessor','CAN'))  RTIBlockInterface=struct('OutputPortsWidth',int32([1 1 1 1]),'OutputPortsActive',[1 1 1 1],'OutputPortsName',{{'Oil_Temperature',['RX status'],['RX time'],['RX delta time']}},'OutputPortsDataType',{{'SS_DOUBLE','SS_DOUBLE','SS_DOUBLE','SS_DOUBLE'}},'OutputPortsLabel',{{'Oil_Temperature','','',''}},'OutputPortsLabelMode','ON','InputPortsWidth',int32(0),'InputPortsActive',0,'DialogFcn','rtican_message_interface_gui','BlockDisplay',{{'','center'}},'IconTransparency','on','ParameterTunableNames',{{}},'InitLevel',3,'BlockName',struct('Token',{{'Oiltemperature'}}),'SampleTime',{{-1}},'TriggerPort',{{'none'}},'EnablePort',{{'none'}})  RTIBlockParameters=struct('BoardTypeNo',{{1,'OFF',[]}},'BoardNo',{{2,'ON',[1 16]}},'ChannelNo',{{1,'ON',[1 2]}},'Parameters',{{struct('DataFileSupport',struct('DataFileSelectedMaster',1,'DataFileSelectedLocal',1,'DataFileName','c:\users\deltaracing\documents\canoe\dr18e\dbc\dr18e.dbc|','DataFileDate',['16-Feb-2019 13:23:09'],'SelectedFile','..\..\..\canoe\dr18e_test\dr18e\dbc\dr18e.dbc','InterfaceFcn','rtican_dbc_file_parser'),'Options',struct('StatusSelected',1,'TimeSelected',1,'DeltaTimeSelected',1,'BytePortSelected',0,'MessageLengthSelected',0,'TriggerPort',struct('Selected',0,'TriggerType',0),'UserCoding',struct('Selected',0,'InterfaceFile','UserDecodingFile','FcnName','UserDecodeFcn','InportSelected',0,'InportWidth',1,'OutportSelected',0,'OutportWidth',1),'EnablePortSelected',0,'SignalOnPortnameSelected',1,'UseRXService',0),'Message',struct('MsgOnBlocknameSelected',1,'MsgName','Oiltemperature','MsgIdFormat',0,'MsgId',792,'MsgLength',2,'NumSignals',1,'SampleTime',-1,'Signal',struct('SgnName','Oil_Temperature','SgnStartBit',0,'SgnLength',16,'ByteLayout',0,'Factor',0.1,'Offset',0,'SgnComment','','SgnUnit','°C','Min',0,'Max',0,'SgnType',0,'SLDataType','SS_DOUBLE','DataType',1,'ModeValue',-1),'MsgIdNumFormat',0,'MsgComment',{{''}}),'Version',1.2,'general',struct('isFromLib',0)),'OFF',[]}},'GroupId',{{struct('Group',{{'RTICAN'}},'No',1,'Behavior',{{'NAMECHANGE'}},'BlockType',{{'SINK'}},'NameChangeFlag',0),'OFF',[]}},'SFcnRTICANMessage',{{struct('MsgType','RX','SFcnPortType','Scalar','MsgName','Oiltemperature','MsgIdFormat','STD','MsgId',792,'MsgLength',2,'NumSignals',1,'SampleTime',-1,'Signal',struct('SgnName','Oil_Temperature','SgnStartBit',0,'SgnLength',16,'ByteLayout',['little endian'],'Factor',0.1,'Offset',0,'SgnType','standard','SLDataType','SS_DOUBLE','DataType',['signed int'],'ModeValue',-1),'StatusSelected','yes','TimeSelected','yes','DeltaTimeSelected','yes','BytePortSelected','no','MessageLengthSelected','no','TriggerPort',struct('Selected','no','TriggerType',0),'UserCoding',struct('Selected','no','InterfaceFile','UserDecodingFile','FcnName','UserDecodeFcn','InportSelected','no','InportWidth',1,'OutportSelected','no','OutportWidth',1),'EnablePortSelected','no','UseRXService','no','BoardType','DS1','BoardNo',2,'ControllerNo',1),'OFF',[]}},'TLCFileName',{{'rtican_rx_message','OFF',[]}})  RTISFcnParameters=struct('SFcnRTICANMessage','struct','TLCFileName','char')  RTIBlockParaDefault=struct('BoardTypeNo',4302,'BoardNo',1,'ChannelNo',1,'Parameters',struct('DataFileSupport',struct('DataFileSelectedMaster',0,'DataFileSelectedLocal',0,'DataFileName','','DataFileDate','','SelectedFile',['<no file selected>']),'Options',struct('StatusSelected',1,'TimeSelected',1,'DeltaTimeSelected',1,'BytePortSelected',0,'MessageLengthSelected',0,'TriggerPort',struct('Selected',0,'TriggerType','rising'),'UserCoding',struct('Selected',0,'InterfaceFile','UserDecodingFile','FcnName','UserDecodeFcn','InportSelected',0,'InportWidth',1,'OutportSelected',0,'OutportWidth',1),'EnablePortSelected',0,'SignalOnPortnameSelected',1,'UseRXService',0),'Message',struct('MsgOnBlocknameSelected',0,'MsgName',['RX Message'],'MsgIdFormat',0,'MsgId',100,'MsgLength',8,'NumSignals',1,'SampleTime',-1,'Signal',struct('SgnName',['RX signal'],'SgnStartBit',0,'SgnLength',8,'SgnType',0,'ModeValue',-1,'DataType',0,'SLDataType','SS_DOUBLE','ByteLayout',0,'Factor',1,'Offset',0,'Min',0,'Max',255,'SgnComment',{{}},'SgnUnit',''),'MsgIdNumFormat',0,'MsgComment',{{''}}),'Version',1.2,'general',struct('isFromLib',1)),'GroupId',struct('Group',{{'RTICAN'}},'No',1,'Behavior',{{'NAMECHANGE'}},'BlockType',{{'SINK'}},'NameChangeFlag',0),'SFcnRTICANMessage',struct('MsgType','RX','MsgName',['RX Message'],'MsgIdFormat','STD','MsgId',100,'MsgLength',8,'NumSignals',1,'SampleTime',-1,'Signal',struct('SgnName',['RX signal'],'SgnStartBit',0,'SgnLength',8,'SgnType','standard','ModeValue',-1,'DataType',['unsigned int'],'ByteLayout',['little endian'],'SLDataType','SS_DOUBLE','Factor',1,'Offset',0),'StatusSelected','yes','TimeSelected','yes','DeltaTimeSelected','yes','BytePortSelected','no','MessageLengthSelected','no','EnablePortSelected','no','UserCoding',struct('Selected','no','InterfaceFile','UserDecodingFile','FcnName','UserDecodeFcn','InportSelected','no','InportWidth',1,'OutportSelected','no','OutportWidth',1),'TriggerPort',struct('Selected','no','TriggerType','rising'),'UseRXService','no','BoardType','DS4302','BoardNo',1,'ControllerNo',1,'SFcnPortType','Scalar'),'TLCFileName','rtican_rx_message')
      settings: AttributesFormatString=Group Id: RTICAN1\n  SourceProductName=dSPACE RTI CAN Blockset
  Sensor_Watertemp : rtican/RTICAN Receive (RX)   Reserved1=[]  Reserved2=[]  Reserved3=[]  Reserved4=[]  SfcnMessage=[]  Msg_Struct=[]  BoardTypeNo=[]  BoardNo=[]  ChannelNo=[]  Parameters=[]  DialogFcn=[]  UnitName=[]  Revision=[]  UnitValues=[]  DSProperties=struct('RTI',struct('Version',uint32(5),'BlockType',struct('isSLSource',uint8(1),'isSLSink',uint8(1),'isHWSource',uint8(0),'isHWSink',uint8(0),'isSetup',uint8(0),'isInline',uint8(1),'isNonInline',uint8(0),'isInterrupt',uint8(0),'isChannelwise',uint8(0)),'IOBoardType','RTICAN','UnitType','MESSAGE','Identifier','RX','DialogType','MSVC','BlockSet','RTICAN','SlaveProcessor','CAN'))  RTIBlockInterface=struct('OutputPortsWidth',int32([1 1 1 1 1]),'OutputPortsActive',[1 1 1 1 1],'OutputPortsName',{{'Water_Temperature_Pump','Water_Temperature_Cooler',['RX status'],['RX time'],['RX delta time']}},'OutputPortsDataType',{{'SS_DOUBLE','SS_DOUBLE','SS_DOUBLE','SS_DOUBLE','SS_DOUBLE'}},'OutputPortsLabel',{{'Water_Temperature_Pump','Water_Temperature_Cooler','','',''}},'OutputPortsLabelMode','ON','InputPortsWidth',int32(0),'InputPortsActive',0,'DialogFcn','rtican_message_interface_gui','BlockDisplay',{{'','center'}},'IconTransparency','on','ParameterTunableNames',{{}},'InitLevel',3,'BlockName',struct('Token',{{'Sensor_Watertemp'}}),'SampleTime',{{-1}},'TriggerPort',{{'none'}},'EnablePort',{{'none'}})  RTIBlockParameters=struct('BoardTypeNo',{{1,'OFF',[]}},'BoardNo',{{2,'ON',[1 16]}},'ChannelNo',{{1,'ON',[1 2]}},'Parameters',{{struct('DataFileSupport',struct('DataFileSelectedMaster',1,'DataFileSelectedLocal',1,'DataFileName','c:\users\deltaracing\documents\canoe\dr18e\dbc\dr18e.dbc|','DataFileDate',['16-Feb-2019 13:23:09'],'SelectedFile','..\..\..\canoe\dr18e_test\dr18e\dbc\dr18e.dbc','InterfaceFcn','rtican_dbc_file_parser'),'Options',struct('StatusSelected',1,'TimeSelected',1,'DeltaTimeSelected',1,'BytePortSelected',0,'MessageLengthSelected',0,'TriggerPort',struct('Selected',0,'TriggerType',0),'UserCoding',struct('Selected',0,'InterfaceFile','UserDecodingFile','FcnName','UserDecodeFcn','InportSelected',0,'InportWidth',1,'OutportSelected',0,'OutportWidth',1),'EnablePortSelected',0,'SignalOnPortnameSelected',1,'UseRXService',0),'Message',struct('MsgOnBlocknameSelected',1,'MsgName','Sensor_Watertemp','MsgIdFormat',0,'MsgId',790,'MsgLength',4,'NumSignals',2,'SampleTime',-1,'Signal',struct('SgnName',{'Water_Temperature_Pump','Water_Temperature_Cooler'},'SgnStartBit',{0,16},'SgnLength',{16,16},'ByteLayout',{0,0},'Factor',{0.1,0.1},'Offset',{0,0},'SgnComment',{'',''},'SgnUnit',{'°C','°C'},'Min',{0,0},'Max',{0,0},'SgnType',{0,0},'SLDataType',{'SS_DOUBLE','SS_DOUBLE'},'DataType',{1,1},'ModeValue',{-1,-1}),'MsgIdNumFormat',0,'MsgComment',{{''}}),'Version',1.2,'general',struct('isFromLib',0)),'OFF',[]}},'GroupId',{{struct('Group',{{'RTICAN'}},'No',1,'Behavior',{{'NAMECHANGE'}},'BlockType',{{'SINK'}},'NameChangeFlag',0),'OFF',[]}},'SFcnRTICANMessage',{{struct('MsgType','RX','SFcnPortType','Scalar','MsgName','Sensor_Watertemp','MsgIdFormat','STD','MsgId',790,'MsgLength',4,'NumSignals',2,'SampleTime',-1,'Signal',struct('SgnName',{'Water_Temperature_Pump','Water_Temperature_Cooler'},'SgnStartBit',{0,16},'SgnLength',{16,16},'ByteLayout',{['little endian'],['little endian']},'Factor',{0.1,0.1},'Offset',{0,0},'SgnType',{'standard','standard'},'SLDataType',{'SS_DOUBLE','SS_DOUBLE'},'DataType',{['signed int'],['signed int']},'ModeValue',{-1,-1}),'StatusSelected','yes','TimeSelected','yes','DeltaTimeSelected','yes','BytePortSelected','no','MessageLengthSelected','no','TriggerPort',struct('Selected','no','TriggerType',0),'UserCoding',struct('Selected','no','InterfaceFile','UserDecodingFile','FcnName','UserDecodeFcn','InportSelected','no','InportWidth',1,'OutportSelected','no','OutportWidth',1),'EnablePortSelected','no','UseRXService','no','BoardType','DS1','BoardNo',2,'ControllerNo',1),'OFF',[]}},'TLCFileName',{{'rtican_rx_message','OFF',[]}})  RTISFcnParameters=struct('SFcnRTICANMessage','struct','TLCFileName','char')  RTIBlockParaDefault=struct('BoardTypeNo',4302,'BoardNo',1,'ChannelNo',1,'Parameters',struct('DataFileSupport',struct('DataFileSelectedMaster',0,'DataFileSelectedLocal',0,'DataFileName','','DataFileDate','','SelectedFile',['<no file selected>']),'Options',struct('StatusSelected',1,'TimeSelected',1,'DeltaTimeSelected',1,'BytePortSelected',0,'MessageLengthSelected',0,'TriggerPort',struct('Selected',0,'TriggerType','rising'),'UserCoding',struct('Selected',0,'InterfaceFile','UserDecodingFile','FcnName','UserDecodeFcn','InportSelected',0,'InportWidth',1,'OutportSelected',0,'OutportWidth',1),'EnablePortSelected',0,'SignalOnPortnameSelected',1,'UseRXService',0),'Message',struct('MsgOnBlocknameSelected',0,'MsgName',['RX Message'],'MsgIdFormat',0,'MsgId',100,'MsgLength',8,'NumSignals',1,'SampleTime',-1,'Signal',struct('SgnName',['RX signal'],'SgnStartBit',0,'SgnLength',8,'SgnType',0,'ModeValue',-1,'DataType',0,'SLDataType','SS_DOUBLE','ByteLayout',0,'Factor',1,'Offset',0,'Min',0,'Max',255,'SgnComment',{{}},'SgnUnit',''),'MsgIdNumFormat',0,'MsgComment',{{''}}),'Version',1.2,'general',struct('isFromLib',1)),'GroupId',struct('Group',{{'RTICAN'}},'No',1,'Behavior',{{'NAMECHANGE'}},'BlockType',{{'SINK'}},'NameChangeFlag',0),'SFcnRTICANMessage',struct('MsgType','RX','MsgName',['RX Message'],'MsgIdFormat','STD','MsgId',100,'MsgLength',8,'NumSignals',1,'SampleTime',-1,'Signal',struct('SgnName',['RX signal'],'SgnStartBit',0,'SgnLength',8,'SgnType','standard','ModeValue',-1,'DataType',['unsigned int'],'ByteLayout',['little endian'],'SLDataType','SS_DOUBLE','Factor',1,'Offset',0),'StatusSelected','yes','TimeSelected','yes','DeltaTimeSelected','yes','BytePortSelected','no','MessageLengthSelected','no','EnablePortSelected','no','UserCoding',struct('Selected','no','InterfaceFile','UserDecodingFile','FcnName','UserDecodeFcn','InportSelected','no','InportWidth',1,'OutportSelected','no','OutportWidth',1),'TriggerPort',struct('Selected','no','TriggerType','rising'),'UseRXService','no','BoardType','DS4302','BoardNo',1,'ControllerNo',1,'SFcnPortType','Scalar'),'TLCFileName','rtican_rx_message')
      settings: AttributesFormatString=Group Id: RTICAN1\n  SourceProductName=dSPACE RTI CAN Blockset
  Terminator_1 : Terminator
  Terminator_6 : Terminator
  Terminator_7 : Terminator
  Transmit OK Detection1 : Subsystem
  Transmit OK Detection3 : Subsystem
  Transmit OK Detection4 : Subsystem
  SensorboardRearOut : Outport
  wires:
  Transmit OK Detection3/1(TX Warn) -> Terminator_6/1
  ES_rear/5 -> Transmit OK Detection3/2(TX delta time)
  ES_rear/3 -> Transmit OK Detection3/1(TX status)
  Transmit OK Detection4/1(TX Warn) -> Terminator_7/1
  Sensor_Watertemp/5 -> Transmit OK Detection4/2(TX delta time)
  Sensor_Watertemp/3 -> Transmit OK Detection4/1(TX status)
  Bus Creator/1 -> SensorboardRearOut/1  "RX_SensorboardRear"
  Gain/1 -> Bus Creator/1  "Notaus_links"
  Gain1/1 -> Bus Creator/2  "Notaus_rechts"
  Transmit OK Detection1/1(TX Warn) -> Terminator_1/1
  Oiltemperature/4 -> Transmit OK Detection1/2(TX delta time)
  Oiltemperature/2 -> Transmit OK Detection1/1(TX status)
  ES_rear/1 -> Gain/1  "Notaus_links"
  ES_rear/2 -> Gain1/1  "Notaus_rechts"
  Sensor_Watertemp/1 -> FlightRecorder1/1(In1), Bus Creator/3  "Water_Temperature_Pump"
  Sensor_Watertemp/2 -> FlightRecorder2/1(In1), Bus Creator/4  "Water_Temperature_Cooler"
  Oiltemperature/1 -> FlightRecorder3/1(In1), Bus Creator/5  "Oil_Temperature"

== system DR18E_Testpult/RTI Data/RTI Data Store ==
  RTI Data Store : Subsystem  mask(RTI_DATA_STORE){}
      mask help:
      | RTI Data Store Block. This block is used by RTI to store internal model dependent data. Deleting this block will result in data loss.
      |
      | NEVER DELETE, COPY, OR MODIFY THIS BLOCK!
      mask Help:
      | RTI Data Store Block. This block is used by RTI to store internal model dependent data. Deleting this block will result in data loss.
      | 
      | NEVER DELETE, COPY, OR MODIFY THIS BLOCK!
      mask Display: text(0.5, 0.5, ' ', 'HorizontalAlignment', 'center');

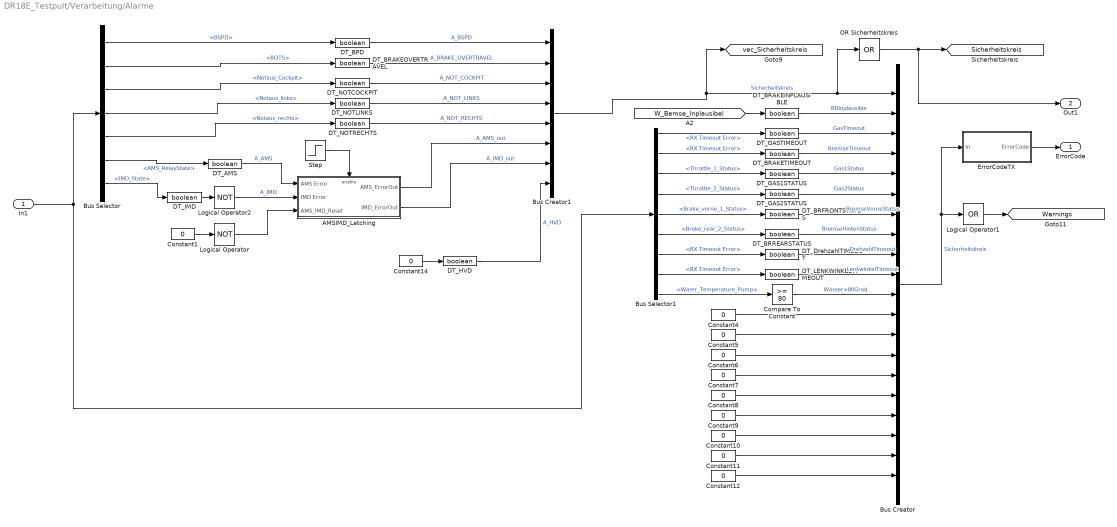
== system DR18E_Testpult/Verarbeitung/Alarme ==
  In1 : Inport
  AMSIMD_Latching : Subsystem
  Bus Creator : BusCreator  Inputs=20
  Bus Creator1 : BusCreator  Inputs=8
  Bus Selector : BusSelector  OutputSignals=RX_SensorboardFront.BSPD,RX_SensorboardFront.BOTS,RX_SensorboardMitte.Notaus_Cockpit,RX_SensorboardRear.Notaus_links,RX_SensorboardRear.Notaus_rechts,BMS_State.AMS_RelayState,RX_CANIO.IMD_State
  Bus Selector1 : BusSelector  OutputSignals=RX_SensorboardFront.RX_Gas.RX Timeout Error,RX_SensorboardFront.RX_Bremse.RX Timeout Error,RX_SensorboardFront.RX_Gas.Throttle_1_Status,RX_SensorboardFront.RX_Gas.Throttle_2_Status,RX_SensorboardFront.RX_Bremse.Brake_vorne_1_Status,RX_SensorboardFront.RX_Bremse.Brake_rear_2_Status,RX_SensorboardMitte.Drehzahlen vorne.RX Timeout Error,RX_Lenkwinkel.RX Timeout Error,RX_SensorboardRear.Water_Temperature_Pump
  Compare To Constant : simulink/Logic and Bit Operations/Compare To Constant  relop=>=  const=80  OutDataTypeStr=boolean
  Constant{1,4..12,14} (11 alike) : Constant  Value=0  OutDataTypeStr=boolean
  DT_AMS : DataTypeConversion  OutDataTypeStr=boolean
  DT_BPD : DataTypeConversion  OutDataTypeStr=boolean
  DT_BRAKEINPLAUSIBLE : DataTypeConversion  OutDataTypeStr=boolean
  DT_BRAKEOVERTRAVEL : DataTypeConversion  OutDataTypeStr=boolean
  DT_BRAKETIMEOUT : DataTypeConversion  OutDataTypeStr=boolean
  DT_BRFRONTSTATUS : DataTypeConversion  OutDataTypeStr=boolean
  DT_BRREARSTATUS : DataTypeConversion  OutDataTypeStr=boolean
  DT_DrehzahlTIMEOUT : DataTypeConversion  OutDataTypeStr=boolean
  DT_GAS1STATUS : DataTypeConversion  OutDataTypeStr=boolean
  DT_GAS2STATUS : DataTypeConversion  OutDataTypeStr=boolean
  DT_GASTIMEOUT : DataTypeConversion  OutDataTypeStr=boolean
  DT_HVD : DataTypeConversion  OutDataTypeStr=boolean
  DT_IMD : DataTypeConversion  OutDataTypeStr=boolean
  DT_LENKWINKELTIMEOUT : DataTypeConversion  OutDataTypeStr=boolean
  DT_NOTCOCKPIT : DataTypeConversion  OutDataTypeStr=boolean
  DT_NOTLINKS : DataTypeConversion  OutDataTypeStr=boolean
  DT_NOTRECHTS : DataTypeConversion  OutDataTypeStr=boolean
  ErrorCodeTX : Subsystem
  Logical Operator : Logic  Operator=NOT  AllPortsSameDT=off  OutDataTypeStr=boolean
  Logical Operator1 : Logic  Operator=OR  Inputs=1  AllPortsSameDT=off  OutDataTypeStr=boolean
  Logical Operator2 : Logic  Operator=NOT  AllPortsSameDT=off  OutDataTypeStr=boolean
  OR Sicherheitskreis : Logic  Operator=OR  Inputs=1  AllPortsSameDT=off  OutDataTypeStr=boolean
  Step : Step  Time=5  SampleTime=0
  ErrorCode : Outport
  Out1 : Outport  Port=2
  tag scope: Sicherheitskreis=global, Warnings=global, vec_Sicherheitskreis=global
  wires:
  Bus Selector/2 -> DT_BRAKEOVERTRAVEL/1  "<BOTS>"
  Bus Selector/3 -> DT_NOTCOCKPIT/1  "<Notaus_Cockpit>"
  Compare To Constant/1 -> Bus Creator/11  "Wasser>80Grad"
  Constant4/1 -> Bus Creator/12
  Constant5/1 -> Bus Creator/13
  Constant6/1 -> Bus Creator/14
  Constant7/1 -> Bus Creator/15
  Constant8/1 -> Bus Creator/16
  Constant9/1 -> Bus Creator/17
  Constant10/1 -> Bus Creator/18
  Constant11/1 -> Bus Creator/19
  Constant12/1 -> Bus Creator/20
  Bus Creator1/1 -> [vec_Sicherheitskreis], OR Sicherheitskreis/1, Bus Creator/1  "Sicherheitskreis"
  DT_BPD/1 -> Bus Creator1/1  "A_BSPD"
  DT_BRAKEOVERTRAVEL/1 -> Bus Creator1/2  "A_BRAKE_OVERTRAVEL"
  DT_NOTCOCKPIT/1 -> Bus Creator1/3  "A_NOT_COCKPIT"
  DT_NOTLINKS/1 -> Bus Creator1/4  "A_NOT_LINKS"
  DT_NOTRECHTS/1 -> Bus Creator1/5  "A_NOT_RECHTS"
  AMSIMD_Latching/1(AMS_ErrorOut) -> Bus Creator1/6  "A_AMS_out"
  AMSIMD_Latching/2(IMD_ErrorOut) -> Bus Creator1/7  "A_IMD_out"
  OR Sicherheitskreis/1 -> Out1/1, [Sicherheitskreis]
  DT_HVD/1 -> Bus Creator1/8  "A_HVD"
  [W_Bemse_Inplausibel] -> DT_BRAKEINPLAUSIBLE/1
  DT_BRAKEINPLAUSIBLE/1 -> Bus Creator/2  "BRInplausible"
  Bus Creator/1 -> ErrorCodeTX/1(In), Logical Operator1/1  "Sicherheitskreis"
  Logical Operator1/1 -> [Warnings]
  DT_GASTIMEOUT/1 -> Bus Creator/3  "GasTimeout"
  Bus Selector1/2 -> DT_BRAKETIMEOUT/1  "<RX Timeout Error>"
  DT_BRAKETIMEOUT/1 -> Bus Creator/4  "BremseTimeout"
  In1/1 -> Bus Selector1/1, Bus Selector/1
  Bus Selector1/1 -> DT_GASTIMEOUT/1  "<RX Timeout Error>"
  Bus Selector/4 -> DT_NOTLINKS/1  "<Notaus_links>"
  Bus Selector/5 -> DT_NOTRECHTS/1  "<Notaus_rechts>"
  Bus Selector/7 -> DT_IMD/1  "<IMD_State>"
  Bus Selector/6 -> DT_AMS/1  "<AMS_RelayState>"
  Constant14/1 -> DT_HVD/1
  ErrorCodeTX/1(ErrorCode) -> ErrorCode/1
  Bus Selector1/3 -> DT_GAS1STATUS/1  "<Throttle_1_Status>"
  Bus Selector1/4 -> DT_GAS2STATUS/1  "<Throttle_2_Status>"
  Bus Selector1/5 -> DT_BRFRONTSTATUS/1  "<Brake_vorne_1_Status>"
  Bus Selector1/6 -> DT_BRREARSTATUS/1  "<Brake_rear_2_Status>"
  Bus Selector1/7 -> DT_DrehzahlTIMEOUT/1  "<RX Timeout Error>"
  Bus Selector1/8 -> DT_LENKWINKELTIMEOUT/1  "<RX Timeout Error>"
  DT_GAS1STATUS/1 -> Bus Creator/5  "Gas1Status"
  DT_GAS2STATUS/1 -> Bus Creator/6  "Gas2Status"
  DT_BRFRONTSTATUS/1 -> Bus Creator/7  "BremseVorneStatus"
  DT_BRREARSTATUS/1 -> Bus Creator/8  "BremseHintenStatus"
  DT_DrehzahlTIMEOUT/1 -> Bus Creator/9  "DrehzahlTimeout"
  DT_LENKWINKELTIMEOUT/1 -> Bus Creator/10  "LenkwinkelTimeout"
  Bus Selector1/9 -> Compare To Constant/1  "<Water_Temperature_Pump>"
  Bus Selector/1 -> DT_BPD/1  "<BSPD>"
  DT_AMS/1 -> AMSIMD_Latching/1(AMS Error)  "A_AMS"
  DT_IMD/1 -> Logical Operator2/1
  Logical Operator/1 -> AMSIMD_Latching/3(AMS_IMD_Reset)
  Step/1 -> AMSIMD_Latching/Enable
  Constant1/1 -> Logical Operator/1
  Logical Operator2/1 -> AMSIMD_Latching/2(IMD Error)  "A_IMD"
